simulink model "G13_sim_L4"  (R2024b)
settings: Solver=ode23tb  StartTime=0.0  StopTime=0.04  MaxStep=1/fpwm/200  RelTol=1e-3
undefined symbols (not defined in the file): Cf, fpwm, Lf, ri, Rmax, U
libraries: spsSeriesRLCBranchLib x4, spsCurrentMeasurementLib x3, spsVoltageMeasurementLib x3, spsDiodeLib x1, spsMosfetLib x1, spsMeanLib x1, spsDCVoltageSourceLib x1, sps_lib x1
settings Model: Creator=Martinha  LastModifiedBy=franc

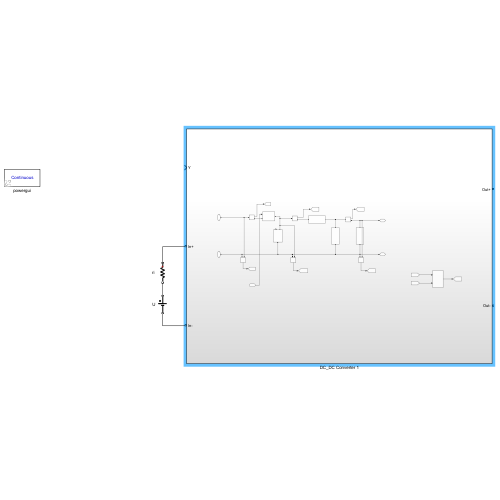
[thumbnail: Simulink's stored preview of the top-level diagram]
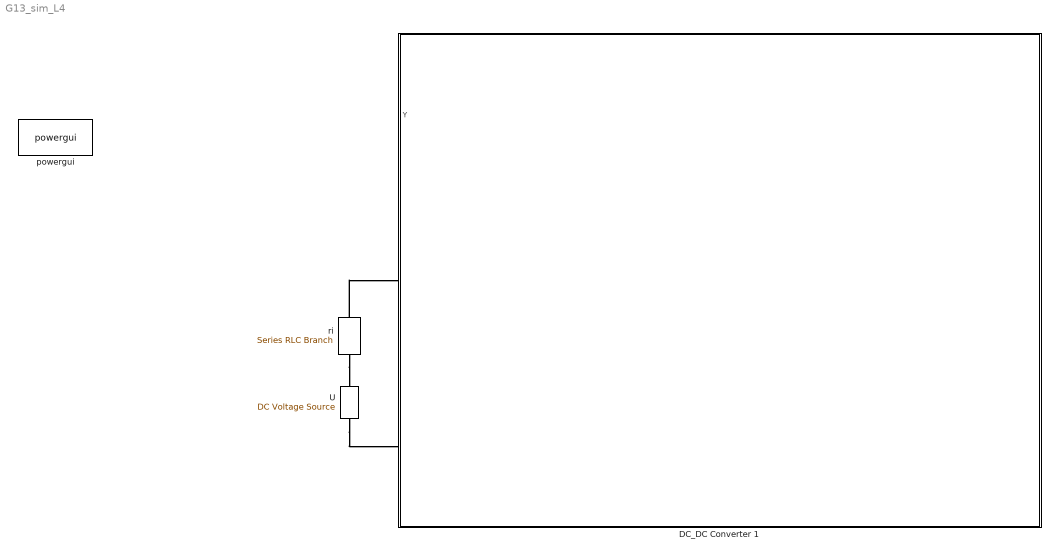
== system G13_sim_L4 ==
  DC_DC Converter 1 : Subsystem
  U : spsDCVoltageSourceLib/DC Voltage Source  Amplitude=U  Measurements=None
  powergui : sps_lib/powergui  Priority=1  SimulationMode=Continuous  SampleTime=50e-6  frequency=60  Iterations=50  frequencyindice=0  Pbase=100e6  ErrMax=1e-4  UnitsV=kV  UnitsW=MW  buscounter=0  FunctionMessages=off  echomessages=off  EnableUseOfTLC=off  CurrentSourceSwitches=off  DisableSnubberDevices=off  DisableRonSwitches=off  DisableVfSwitches=off  DisplayEquations=off  AutomaticDiscreteSolvers=off  SolverType=Tustin/Backward Euler (TBE)  Interpol=off  ExternalGateDelay=off  methode=off  Ts=100  x0status=blocks  SPID=on  SwTol=0  HookPort=off  NonlinearTolerance=1e-4  nMaxIteration=100  ContinueOnMaxIteration=off  RestoreLinks=warning  ResistiveCurrentMeasurement=off  Frange=[0:2:500]  Ylog=off  Xlog=on  ShowGrid=off  save=off  variable=ZData  structure=0  ZoomFFT=off  StartTime=0.0  cycles=1  DisplayStyle=1  fundamental=60  FreqAxis=off  MaxFrequency=1000  frequencyindicesteady=1  RmsSteady=1  display=off
  ri : spsSeriesRLCBranchLib/Series RLC Branch  LConnTagsString=__new0  RConnTagsString=__new0  BranchType=R  Resistance=ri  Inductance=1e-3  SetiL0=off  InitialCurrent=0  Capacitance=1e-6  Setx0=off  InitialVoltage=0  Measurements=None
  connections:
  ri/RConn1 -- U/RConn1
  ri/LConn1 -- DC_DC Converter 1/LConn1
  U/LConn1 -- DC_DC Converter 1/LConn2

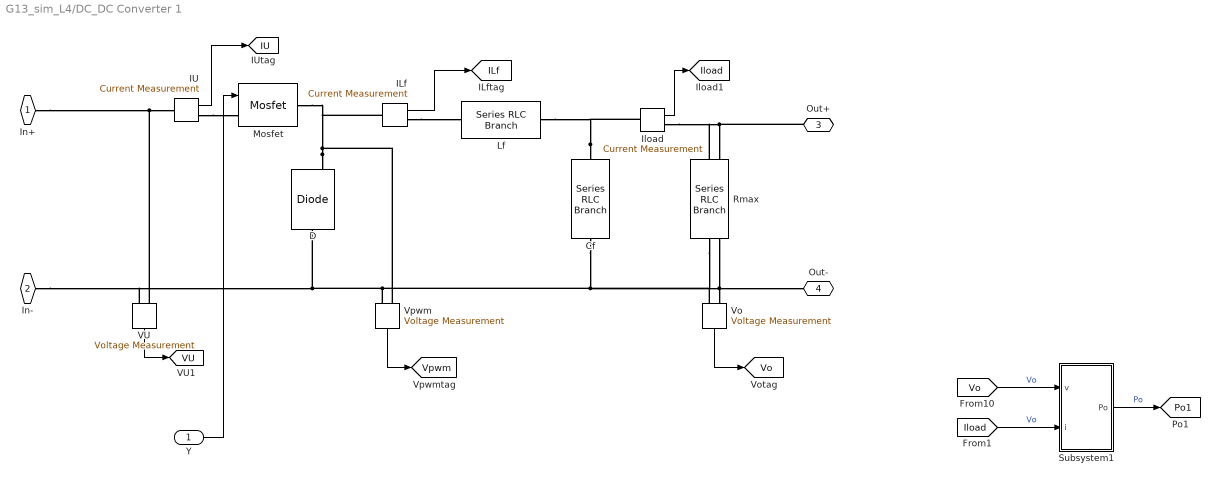
== system G13_sim_L4/DC_DC Converter 1 ==
  Y : Inport
  Cf : spsSeriesRLCBranchLib/Series RLC Branch  LConnTagsString=__new0  RConnTagsString=__new0  BranchType=C  Resistance=1  Inductance=1e-3  SetiL0=off  InitialCurrent=0  Capacitance=Cf  Setx0=on  InitialVoltage=48  Measurements=None
  D : spsDiodeLib/Diode  Ron=Ron  Lon=0  Vf=Vd  IC=0  UseSnubber=0  Rs=Rs  Cs=Cs  Measurements=on
  ILf : spsCurrentMeasurementLib/Current Measurement  PhasorSimulation=off  OutputType=Complex  PSBequivalent=0
  IU : spsCurrentMeasurementLib/Current Measurement  PhasorSimulation=off  OutputType=Complex  PSBequivalent=0
  Iload : spsCurrentMeasurementLib/Current Measurement  PhasorSimulation=off  OutputType=Complex  PSBequivalent=0
  Lf : spsSeriesRLCBranchLib/Series RLC Branch  LConnTagsString=__new0  RConnTagsString=__new0  BranchType=L  Resistance=1  Inductance=Lf  SetiL0=off  InitialCurrent=0  Capacitance=1e-6  Setx0=off  InitialVoltage=0  Measurements=None
  Mosfet : spsMosfetLib/Mosfet  Ron=Ron  Lon=0  Rd=Rdson  Vfd=Vd  IC=0  Rs=Rs  Cs=Cs  Measurements=off
  Rmax : spsSeriesRLCBranchLib/Series RLC Branch  LConnTagsString=__new0  RConnTagsString=__new0  BranchType=R  Resistance=Rmax  Inductance=1e-3  SetiL0=off  InitialCurrent=0  Capacitance=1e-6  Setx0=off  InitialVoltage=0  Measurements=None
  Subsystem1 : Subsystem
  VU : spsVoltageMeasurementLib/Voltage Measurement  PhasorSimulation=off  OutputType=Complex  PSBequivalent=0
  Vo : spsVoltageMeasurementLib/Voltage Measurement  PhasorSimulation=off  OutputType=Complex  PSBequivalent=0
  Vpwm : spsVoltageMeasurementLib/Voltage Measurement  PhasorSimulation=off  OutputType=Complex  PSBequivalent=0
  In+ : PMIOPort  Side=Left
  In- : PMIOPort  Port=2  Side=Left
  Out+ : PMIOPort  Port=3  Side=Right
  Out- : PMIOPort  Port=4  Side=Right
  tag scope: ILf=global, IU=global, Iload=global, Po1=global, VU=global, Vo=global, Vpwm=global
  wires:
  Vpwm/1 -> [Vpwm]
  Vo/1 -> [Vo]
  VU/1 -> [VU]
  Iload/1 -> [Iload]
  Y/1 -> Mosfet/1
  IU/1 -> [IU]
  ILf/1 -> [ILf]
  [Vo] -> Subsystem1/1(v)  "Vo"
  [Iload] -> Subsystem1/2(i)  "Vo"
  Subsystem1/1(Po) -> [Po1]  "Po"
  connections:
  Vo/LConn1 -- Out+/RConn1 -- Rmax/LConn1 -- Iload/RConn1
  Cf/LConn1 -- Lf/RConn1 -- Iload/LConn1
  Cf/RConn1 -- In-/RConn1 -- VU/LConn2 -- D/LConn1 -- Vpwm/LConn2 -- Out-/RConn1 -- Vo/LConn2 -- Rmax/RConn1
  D/RConn1 -- Mosfet/RConn1 -- ILf/LConn1 -- Vpwm/LConn1
  VU/LConn1 -- IU/LConn1 -- In+/RConn1
  IU/RConn1 -- Mosfet/LConn1
  ILf/RConn1 -- Lf/LConn1

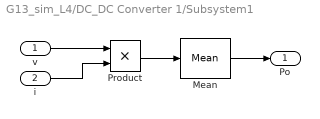
== system G13_sim_L4/DC_DC Converter 1/Subsystem1 ==
  v : Inport
  i : Inport  Port=2
  Mean : spsMeanLib/Mean  Freq=fpwm/10  Vinit=100  Ts=0
  Product : Product
  Po : Outport
  wires:
  Mean/1 -> Po/1
  i/1 -> Product/2
  v/1 -> Product/1
  Product/1 -> Mean/1
